simulink model "untitled"  (R2021b)
settings: Solver=VariableStepAuto  StartTime=0.0  StopTime=10.0  RelTol=1e-3
undefined symbols (not defined in the file or in its folder): C1_lut, C2_lut, crate_bp, DiscIntNeverNeededParam, R0_lut, R1_lut, R2_lut, raptor_get_param_eval, raptor_xcp_function, soc_bp
libraries: arc_dd_lib x12, Raptor_lib x8, arc_specialized_lib x4, simulink x2, arc_logic_lib x2, arc_fault_lib x2
(part 2 of 2)

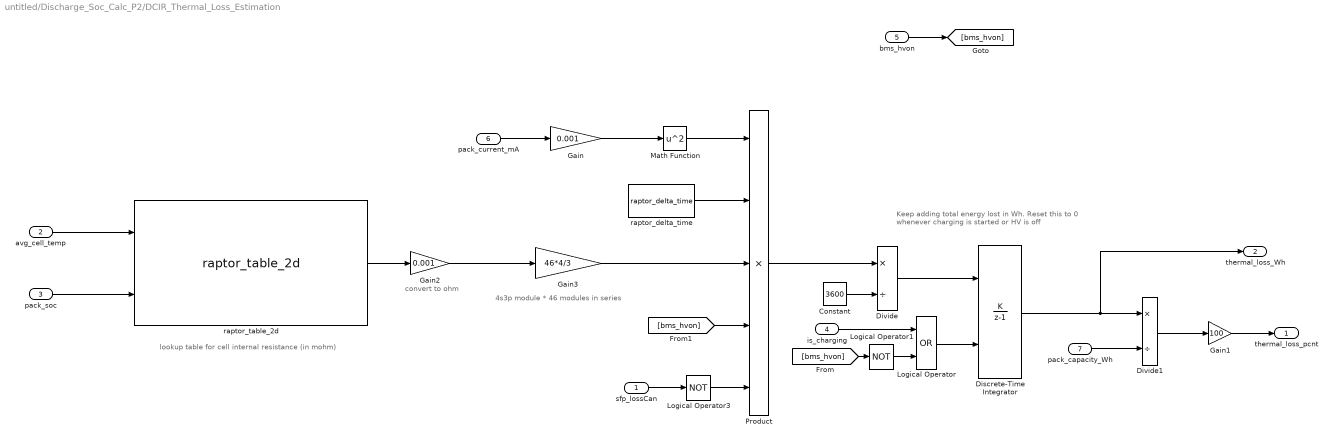
== system untitled/Discharge_Soc_Calc_P2/DCIR_Thermal_Loss_Estimation ==
  note: 4s3p module * 46 modules in series
  note: convert to ohm
  note: lookup table for cell internal resistance (in mohm)
  note: Keep adding total energy lost in Wh. Reset this to 0 whenever charging is started or HV is off
  sfp_lossCan : Inport
  avg_cell_temp : Inport  Port=2
  pack_soc : Inport  Port=3
  is_charging : Inport  Port=4
  bms_hvon : Inport  Port=5
  pack_current_mA : Inport  Port=6
  pack_capacity_Wh : Inport  Port=7
  Constant : Constant  Value=3600
  Discrete-Time Integrator : DiscreteIntegrator  IntegratorMethod=Accumulation: Forward Euler  ExternalReset=level  SampleTime=-1  OutDataTypeStr=single  LimitOutput=on  UpperSaturationLimit=120000  LowerSaturationLimit=0  ICPrevOutput=DiscIntNeverNeededParam  ICPrevScaledInput=DiscIntNeverNeededParam
      settings: AttributesFormatString=|
      | %<UpperSaturationLimit>
      | %<LowerSaturationLimit>
  Divide : Product  Inputs=*/
  Divide1 : Product  Inputs=*/
  Gain : Gain  Gain=0.001
  Gain1 : Gain  Gain=100
  Gain2 : Gain  Gain=0.001
  Gain3 : Gain  Gain=46*4/3
  Logical Operator : Logic  Operator=OR  AllPortsSameDT=off  OutDataTypeStr=boolean
  Logical Operator1 : Logic  Operator=NOT  AllPortsSameDT=off  OutDataTypeStr=boolean
  Logical Operator3 : Logic  Operator=NOT  AllPortsSameDT=off  OutDataTypeStr=boolean
  Math Function : Math  Operator=square  SaturateOnIntegerOverflow=on
  Product : Product  Inputs=5
  raptor_delta_time : Raptor_lib/Triggers/raptor_delta_time  unit=seconds
      settings: SourceProductName=Raptor
  raptor_table_2d : Raptor_lib/Table Lookup/raptor_table_2d  dataName='dcir_p2'  initValue=|  dataType=double  storage=Calibration  initValueX=[5 10 15 20 25 30 35 40 45 50 55 60 65 70 75 80 85 90 95 100]  initValueY=[0 10 25 45]  dataTypeXY=double  storageXY=Calibration  calVisible=on  showTable=off  calGain=1.0  calOffset=0.0  calMax=Inf  calMin=-Inf  calFormat='-1'  calUnit=''  calHelp=''  showBreakpointX=off  dataNameX=[]  calGainX=1.0  calOffsetX=0.0  calMaxX=Inf  calMinX=-Inf  calFormatX='-1'  calUnitX=''  calHelpX=''  showBreakpointY=off  dataNameY=[]  calGainY=1.0  calOffsetY=0.0  calMaxY=Inf  calMinY=-Inf  calFormatY='-1'  calUnitY=''  calHelpY=''  calAccess=1  calFunction=raptor_xcp_function(gcb)  measureEnable=off  mName=[raptor_get_param_eval(gcb,'dataName'), '_Output']
      | [5.77000000000000	5.16400000000000	4.79100000000000	4.55700000000000	4.41700000000000	3.92700000000000	3.85800000000000	3.82300000000000	3.47000000000000	3.46700000000000	3.47200000000000	3.47900000000000	3.48400000000000	3.48600000000000	3.49400000000000	3.51100000000000	3.54500000000000	3.60100000000000	3.73100000000000	4.16700000000000;
      | 2.54900000000000	2.36200000000000	2.27500000000000	2.50700000000000	2.44900000000000	2.31500000000000	2.25000000000000	2.18000000000000	2.18500000000000	2.20700000000000	2.23300000000000	2.24600000000000	2.24200000000000	2.24000000000000	2.24800000000000	2.25000000000000	2.26100000000000	2.28500000000000	2.35800000000000	2.64100000000000;
      | 1.86600000000000	1.67500000000000	1.55200000000000	1.48700000000000	1.42900000000000	1.39400000000000	1.37700000000000	1.35600000000000	1.36400000000000	1.40000000000000	1.44500000000000	1.46200000000000	1.47000000000000	1.46800000000000	1.46100000000000	1.46800000000000	1.47100000000000	1.46800000000000	1.49800000000000	1.68000000000000;
      | 1.27500000000000	1.07800000000000	0.994000000000000	0.934000000000000	0.911000000000000	0.891000000000000	0.880000000000000	0.879000000000000	0.870000000000000	0.877000000000000	0.940000000000000	0.967000000000000	0.967000000000000	0.955000000000000	0.959000000000000	0.958000000000000	0.942000000000000	0.921000000000000	0.920000000000000	1.05600000000000]
      settings: SourceProductName=Raptor
  thermal_loss_pcnt : Outport
  thermal_loss_Wh : Outport  Port=2
  wires:
  pack_current_mA/1 -> Gain/1
  Math Function/1 -> Product/1
  raptor_delta_time/1 -> Product/2
  avg_cell_temp/1 -> raptor_table_2d/1
  pack_soc/1 -> raptor_table_2d/2
  raptor_table_2d/1 -> Gain2/1
  Gain/1 -> Math Function/1
  Product/1 -> Divide/1
  Constant/1 -> Divide/2
  Divide/1 -> Discrete-Time Integrator/1
  Logical Operator/1 -> Discrete-Time Integrator/2
  is_charging/1 -> Logical Operator/1
  Logical Operator1/1 -> Logical Operator/2
  bms_hvon/1 -> [bms_hvon]
  Discrete-Time Integrator/1 -> thermal_loss_Wh/1, Divide1/1
  pack_capacity_Wh/1 -> Divide1/2
  Divide1/1 -> Gain1/1
  Gain1/1 -> thermal_loss_pcnt/1
  [bms_hvon] -> Logical Operator1/1
  [bms_hvon] -> Product/4
  Logical Operator3/1 -> Product/5
  sfp_lossCan/1 -> Logical Operator3/1
  Gain2/1 -> Gain3/1
  Gain3/1 -> Product/3
